simulink model "pil_target_mpc8610"  (R2023b)
settings: Solver=FixedStepDiscrete  StartTime=0.0  StopTime=10.0  RelTol=1e-3  EnableMultiTasking=on
undefined symbols (not defined in the file or in its folder): Newton, Raphson
settings Model: Creator=mbussjaeger  LastModifiedBy=csax
settings SolverCC: AlgebraicLoopSolver=TrustRegion
settings DataIOCC: LimitDataPoints=on  SaveFormat=Array  SignalLoggingSaveFormat=ModelDataLogs  ReturnWorkspaceOutputs=off
settings OptimizationCC: DefaultParameterBehavior=Inlined  EnhancedBackFolding=on  PassReuseOutputArgsAs=Individual arguments  ExpressionDepthLimit=2147483647  ZeroExternalMemoryAtStartup=off  ZeroInternalMemoryAtStartup=off  OptimizeBlockOrder=speed  DifferentSizesBufferReuse=on  OptimizationCustomize=off  EfficientTunableParamExpr=on
settings DebuggingCC: UnderspecifiedInitializationDetection=Classic  MergeDetectMultiDrivingBlocksExec=none  SolverPrmCheckMsg=warning  ParameterTunabilityLossMsg=error  FcnCallInpInsideContextMsg=warning  UnconnectedInputMsg=warning  UnconnectedOutputMsg=warning  UnconnectedLineMsg=warning  AllowSymbolicDim=off  StateNameClashWarn=warning  SFUnexpectedBacktrackingDiag=warning  SFNoUnconditionalDefaultTransitionDiag=warning  SFExecutionAtInitializationDiag=none  ArithmeticOperatorsInVariantConditions=warning
settings HardwareCC: ProdBitPerPointer=32  ProdBitPerSizeT=32  ProdBitPerPtrDiffT=32  ProdLargestAtomicInteger=Long  ProdLargestAtomicFloat=Double  ProdEndianess=BigEndian  ProdWordSize=32  ProdHWDeviceType=Freescale->MPC86xx
settings ModelReferenceCC: EnableRefExpFcnMdlSchedulingChecks=on  PropagateSignalLabelsOutOfModel=off
settings SFSimCC: SimUseLocalCustomCode=off  MATLABDynamicMemAlloc=off  CustomCodeUndefinedFunction=UseInterfaceOnly
settings RTWCC: Description=Embedded Coder  SystemTargetFile=ert.tlc  TemplateMakefile=ert_default_tmf  RTWUseLocalCustomCode=off  Toolchain=TRACE32 XIL Diab Compiler Power Architecture | gmake makefile
settings CodeAppCC: ForceParamTrailComments=on  IgnoreCustomStorageClasses=off  MaxIdLength=63  OperatorAnnotations=on  SimulinkDataObjDesc=on  SFDataObjDesc=on  InsertBlockDesc=on
settings ERTTargetCC: GenerateSampleERTMain=on  InlinedParameterPlacement=NonHierarchical  ERTCustomFileTemplate=example_file_process.tlc
settings ConfigComp: CovMetricSettings=dw  CovSaveCumulativeToWorkspaceVar=on  CovSaveSingleToWorkspaceVar=on  CovExternalEMLEnable=off  CovSFcnEnable=off

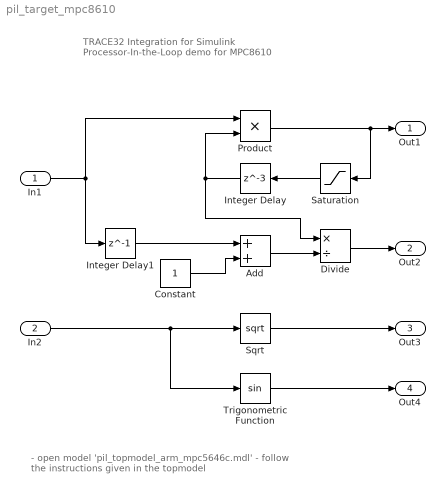
== system pil_target_mpc8610 ==
  note: TRACE32 Integration for Simulink
      | Processor-In-the-Loop demo for MPC8610
  note: - open model 'pil_topmodel_arm_mpc5646c.mdl'
      | - follow the instructions given in the topmodel
  In1 : Inport  OutDataTypeStr=uint16
  In2 : Inport  Port=2  OutDataTypeStr=single
  Add : Sum  AccumDataTypeStr=uint16
  Constant : Constant  OutDataTypeStr=uint16
  Divide : Product  Inputs=*/  OutDataTypeStr=uint16
  Integer Delay : Delay  DelayLength=3
  Integer Delay1 : Delay  DelayLength=1
  Product : Product  OutDataTypeStr=uint16  RndMeth=Zero
  Saturation : Saturate  UpperLimit=6550  LowerLimit=1
  Sqrt : Sqrt  AlgorithmType=Newton-Raphson
  Trigonometric Function : Trigonometry
  Out1 : Outport  OutDataTypeStr=uint16
  Out2 : Outport  Port=2  OutDataTypeStr=uint16
  Out3 : Outport  Port=3
  Out4 : Outport  Port=4
  wires:
  In1/1 -> Product/1, Integer Delay1/1
  Saturation/1 -> Integer Delay/1
  Integer Delay/1 -> Product/2, Divide/1
  Product/1 -> Saturation/1, Out1/1
  Divide/1 -> Out2/1
  In2/1 -> Trigonometric Function/1, Sqrt/1
  Sqrt/1 -> Out3/1
  Trigonometric Function/1 -> Out4/1
  Add/1 -> Divide/2
  Constant/1 -> Add/2
  Integer Delay1/1 -> Add/1
